simulink model "motorsystem"  (R2024b)
settings: Solver=VariableStepAuto  StartTime=0.0  StopTime=15  RelTol=1e-3
undefined symbols (not defined in the file): b, J, ke, kt, L, R
settings Model: Creator=omari  LastModifiedBy=omari

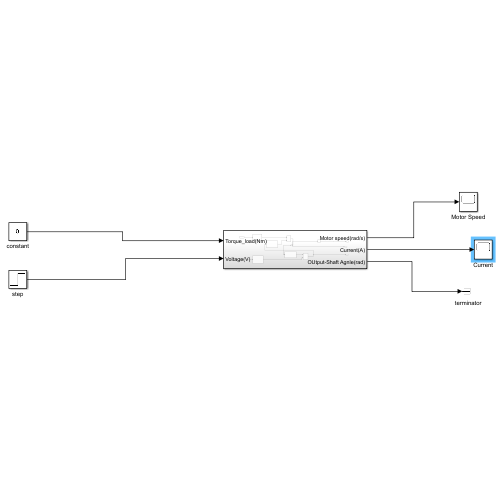
[thumbnail: Simulink's stored preview of the top-level diagram]
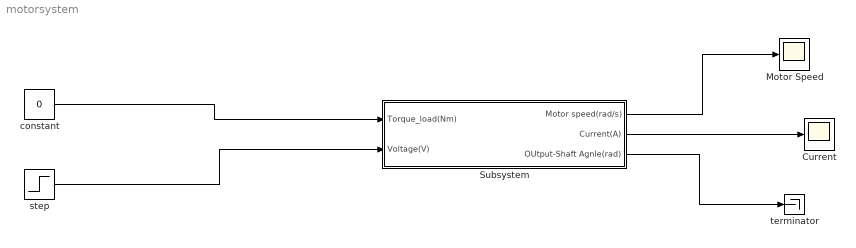
== system motorsystem ==
  Current : Scope
  Motor Speed : Scope
  Subsystem : Subsystem
  constant : Constant  Value=0
  step : Step  Time=6  After=12  SampleTime=0
  terminator : Terminator
  wires:
  step/1 -> Subsystem/2(Voltage(V))
  constant/1 -> Subsystem/1(Torque_load(Nm))
  Subsystem/3(OUtput-Shaft Agnle(rad)) -> terminator/1
  Subsystem/2(Current(A)) -> Current/1
  Subsystem/1(Motor speed(rad/s)) -> Motor Speed/1

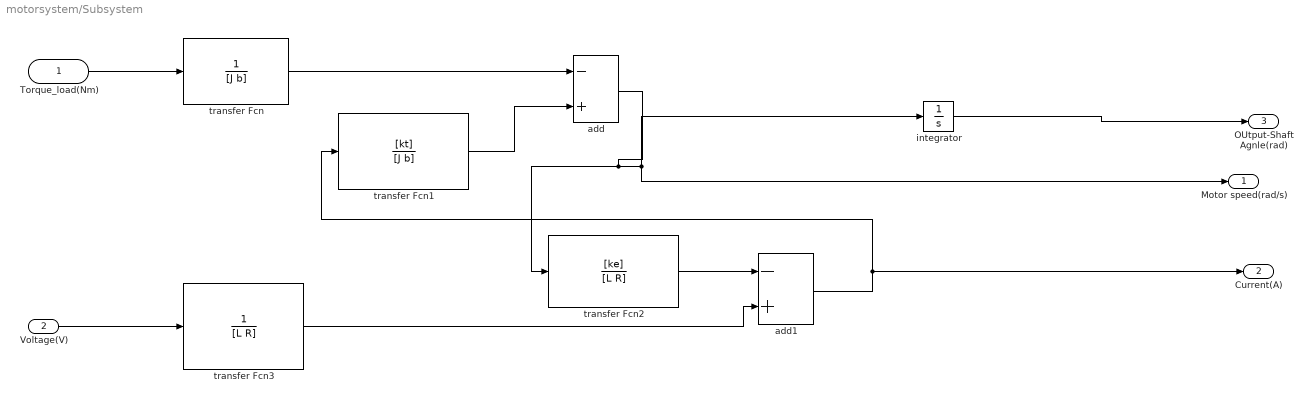
== system motorsystem/Subsystem ==
  Torque_load(Nm) : Inport
  Voltage(V) : Inport  Port=2
  add : Sum  Inputs=-+
  add1 : Sum  Inputs=-+
  integrator : Integrator
  transfer Fcn : TransferFcn  Denominator=[J b]
  transfer Fcn1 : TransferFcn  Numerator=[kt]  Denominator=[J b]
  transfer Fcn2 : TransferFcn  Numerator=[ke]  Denominator=[L R]
  transfer Fcn3 : TransferFcn  Denominator=[L R]
  Motor speed(rad/s) : Outport
  Current(A) : Outport  Port=2
  OUtput-Shaft Agnle(rad) : Outport  Port=3
  wires:
  add/1 -> transfer Fcn2/1, Motor speed(rad/s)/1, integrator/1
  add1/1 -> Current(A)/1, transfer Fcn1/1
  Torque_load(Nm)/1 -> transfer Fcn/1
  transfer Fcn3/1 -> add1/2
  transfer Fcn2/1 -> add1/1
  Voltage(V)/1 -> transfer Fcn3/1
  transfer Fcn/1 -> add/1
  transfer Fcn1/1 -> add/2
  integrator/1 -> OUtput-Shaft Agnle(rad)/1
